simulink subsystem "VehicleBody1DOFLongitudinalSSC"  (R2024a)
settings: Solver=VariableStepAuto  StartTime=0.0  StopTime=10.0  RelTol=1e-3
undefined symbols (not defined in the file): BdyFrm, EnvGrvty, InertFrm, PlntVehCGHgtAxl, PlntVehHtchDst, PlntVehHtchHgtAxl, PlntVehHtchLatDst, PlntWhlLdRadius
libraries: nesl_utility_internal x5, sdl_lib x1
settings Model: ModifiedByFormat=The MathWorks, Inc.  Creator=The MathWorks, Inc.  LastModifiedBy=The MathWorks, Inc.
settings OptimizationCC: ReuseModelBlockBuffer=off
settings DebuggingCC: SubsystemReferenceDiagnosticForUnitTest=warning
settings RTWCC: GPUComputeCapability=3.5

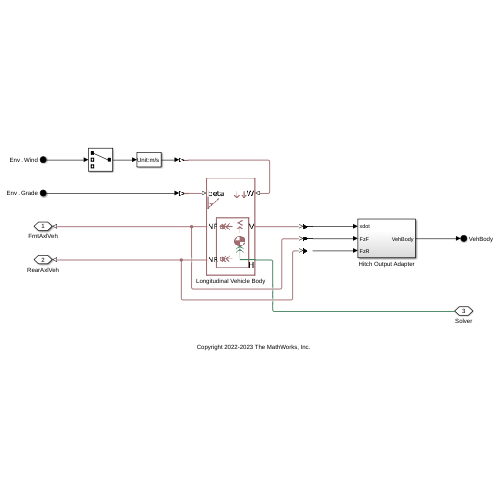
[thumbnail: Simulink's stored preview of the top-level diagram]
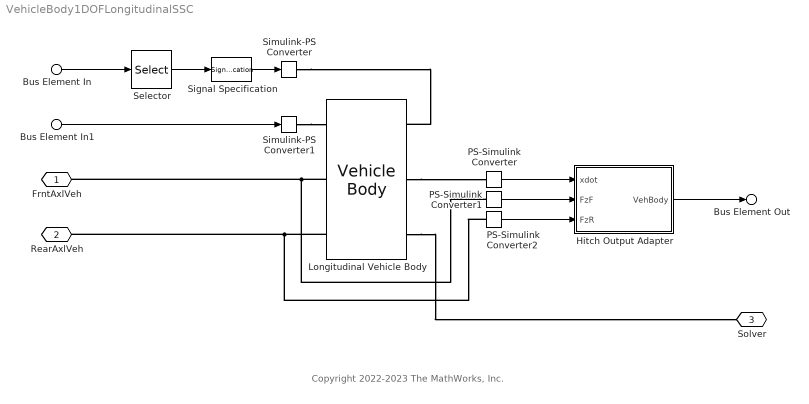
== system VehicleBody1DOFLongitudinalSSC ==
  note: Copyright 2022-2023 The MathWorks, Inc.
  Bus Element In : Inport  PortName=Env  Element=Wind
  Bus Element In1 : Inport  PortName=Env  Element=Grade
  Hitch Output Adapter : Subsystem
  Longitudinal Vehicle Body : sdl_lib/Tires & Vehicles/Vehicle Body  mass=PlntVehMass kg  n_w=PlntVehNumWhlFrntAxl  x_f=PlntVehDstCGFrntAxl m  x_r=PlntVehDstCGRearAxl m  y_c=PlntVehCGHgtAxl+PlntWhlLdRadius m  mass_var=simscape.enum.onoff.off  g=EnvGrvty m/s^2  liftoff_warning=simscape.enum.onoff.off  area=PlntVehAeroFrntArea m^2  Cd=PlntVehAeroDragCff  rho=EnvAirDen kg/m^3  model_pitch=simscape.enum.onoff.off  inertia=PlntVehPitchMomentInertia kg*m^2  suspension_model=sdl.enum.linearTLU.linear  k_f=PlntVeh3DOFFrntSuspStiff N/m  b_f=PlntVeh3DOFFrntSuspDamp N*s/m  k_r=PlntVeh3DOFRearSuspStiff N/m  b_r=PlntVeh3DOFRearSuspDamp N*s/m  k_f_TLU=[-2000, -1000, 0, 1000, 2000] N  x_f_TLU=[-.4, -.2, 0, .2, .4] m  b_f_TLU=[-200, -100, 0, 100, 200] N  v_f_TLU=[-4, -2, 0, 2, 4] m/s  k_r_TLU=[-2000, -1000, 0, 1000, 2000] N  x_r_TLU=[-.4, -.2, 0, .2, .4] m  b_r_TLU=[-200, -100, 0, 100, 200] N  v_r_TLU=[-4, -2, 0, 2, 4] m/s  interp_method=simscape.enum.interpolation.linear  extrap_method=simscape.enum.extrapolation.linear  model_hardstop=simscape.enum.onoff.off  upper_bound_f=.25 m  lower_bound_f=-.25 m  stop_k_f=1e6 N/m  stop_b_f=150 N*s/m  upper_bound_r=.25 m  lower_bound_r=-.25 m  stop_k_r=1e6 N/m  stop_b_r=150 N*s/m  initial_pitch=PlntVehInitPitchAng rad  initial_pitch_rate=PlntVehInitPitchRate rad/s  v_specify=off  v_priority=High  v=0 m/s  v_nominal_specify=off  v_nominal_value=1  v_nominal_unit=m/s
  PS-Simulink Converter : nesl_utility_internal/PS-Simulink Converter  PhysicalDomain=network_engine_domain  SubClassName=ps_output  LeftPortType=input  RightPortType=output  PseudoPeriodic=off  Frequencies=[]  VectorFormat=inherit  Unit=inherit  AffineConversion=off
  PS-Simulink Converter1 : nesl_utility_internal/PS-Simulink Converter  PhysicalDomain=network_engine_domain  SubClassName=ps_output  LeftPortType=input  RightPortType=output  PseudoPeriodic=off  Frequencies=[]  VectorFormat=inherit  Unit=inherit  AffineConversion=off
  PS-Simulink Converter2 : nesl_utility_internal/PS-Simulink Converter  PhysicalDomain=network_engine_domain  SubClassName=ps_output  LeftPortType=input  RightPortType=output  PseudoPeriodic=off  Frequencies=[]  VectorFormat=inherit  Unit=inherit  AffineConversion=off
  Selector : Selector  InputPortWidth=3  IndexOptions=Index vector (dialog)  Indices=[1]  OutputSizes=1
  Signal Specification : SignalSpecification  Unit=m/s
  Simulink-PS Converter : nesl_utility_internal/Simulink-PS Converter  PhysicalDomain=network_engine_domain  SubClassName=ps_input  LeftPortType=input  RightPortType=output  PseudoPeriodic=off  Frequencies=[]  NoiseDistribution=none  NoiseParameters=[]  Unit=m/s  AffineConversion=off  FilteringAndDerivatives=provide  SimscapeFilterOrder=1  InputFilterTimeConstant=0.001  UdotUserProvided=0
  Simulink-PS Converter1 : nesl_utility_internal/Simulink-PS Converter  PhysicalDomain=network_engine_domain  SubClassName=ps_input  LeftPortType=input  RightPortType=output  PseudoPeriodic=off  Frequencies=[]  NoiseDistribution=none  NoiseParameters=[]  Unit=deg  AffineConversion=off  FilteringAndDerivatives=provide  SimscapeFilterOrder=1  InputFilterTimeConstant=0.001  UdotUserProvided=0
  FrntAxlVeh : PMIOPort  Side=Left
  RearAxlVeh : PMIOPort  Port=2  Side=Left
  Solver : PMIOPort  Port=3  Side=Right
  Bus Element Out : Outport  PortName=VehBody
  wires:
  Bus Element In/1 -> Selector/1
  PS-Simulink Converter/1 -> Hitch Output Adapter/1(xdot)
  Selector/1 -> Signal Specification/1
  Bus Element In1/1 -> Simulink-PS Converter1/1
  PS-Simulink Converter2/1 -> Hitch Output Adapter/3(FzR)
  PS-Simulink Converter1/1 -> Hitch Output Adapter/2(FzF)
  Signal Specification/1 -> Simulink-PS Converter/1
  Hitch Output Adapter/1(VehBody) -> Bus Element Out/1
  connections:
  Longitudinal Vehicle Body/RConn2 -- PS-Simulink Converter1/LConn1 -- FrntAxlVeh/RConn1
  Longitudinal Vehicle Body/RConn1 -- PS-Simulink Converter2/LConn1 -- RearAxlVeh/RConn1
  Longitudinal Vehicle Body/LConn2 -- PS-Simulink Converter/LConn1
  Longitudinal Vehicle Body/LConn1 -- Solver/RConn1
  Simulink-PS Converter/RConn1 -- Longitudinal Vehicle Body/LConn3
  Simulink-PS Converter1/RConn1 -- Longitudinal Vehicle Body/RConn3

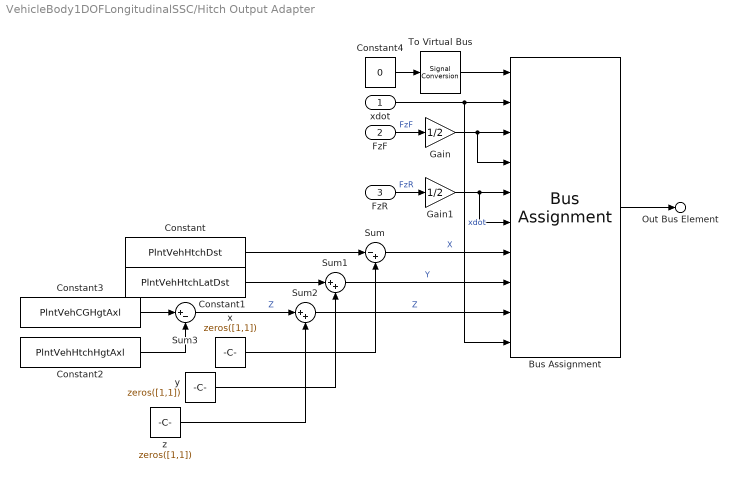
== system VehicleBody1DOFLongitudinalSSC/Hitch Output Adapter ==
  xdot : Inport
  FzF : Inport  Port=2
  FzR : Inport  Port=3
  Bus Assignment : BusAssignment  AssignedSignals=BdyFrm.Cg.Vel.xdot,BdyFrm.Forces.FrntAxl.Lft.Fz,BdyFrm.Forces.FrntAxl.Rght.Fz,BdyFrm.Forces.RearAxl.Lft.Fz,BdyFrm.Forces.RearAxl.Rght.Fz,InertFrm.Hitch.Disp.X,InertFrm.Hitch.Disp.Y,InertFrm.Hitch.Disp.Z,InertFrm.Hitch.Vel.Xdot
  Constant : Constant  Value=PlntVehHtchDst  SampleTime=-1
  Constant1 : Constant  Value=PlntVehHtchLatDst  SampleTime=-1
  Constant2 : Constant  Value=PlntVehHtchHgtAxl  SampleTime=-1
  Constant3 : Constant  Value=PlntVehCGHgtAxl  SampleTime=-1
  Constant4 : Constant  Value=0  OutDataTypeStr=Bus: VehBodyBUS  SampleTime=Inf
  Gain : Gain  Gain=1/2
  Gain1 : Gain  Gain=1/2
  Sum : Sum  Inputs=|-+
  Sum1 : Sum  Inputs=|++
  Sum2 : Sum  Inputs=|++
  Sum3 : Sum  Inputs=|+-
  To Virtual Bus : SignalConversion  ConversionOutput=Virtual bus  OverrideOpt=off
  x : Constant  Value=zeros([1,1])  SampleTime=-1
  y : Constant  Value=zeros([1,1])  SampleTime=-1
  z : Constant  Value=zeros([1,1])  SampleTime=-1
  Out Bus Element : Outport  PortName=VehBody
  wires:
  To Virtual Bus/1 -> Bus Assignment/1
  Bus Assignment/1 -> Out Bus Element/1
  Gain1/1 -> Bus Assignment/5, Bus Assignment/6
  Gain/1 -> Bus Assignment/3, Bus Assignment/4
  FzR/1 -> Gain1/1  "FzR"
  FzF/1 -> Gain/1  "FzF"
  xdot/1 -> Bus Assignment/2, Bus Assignment/10  "xdot"
  Constant4/1 -> To Virtual Bus/1
  z/1 -> Sum2/2
  x/1 -> Sum/2
  y/1 -> Sum1/2
  Constant/1 -> Sum/1
  Sum3/1 -> Sum2/1  "Z"
  Constant3/1 -> Sum3/1
  Sum2/1 -> Bus Assignment/9  "Z"
  Constant2/1 -> Sum3/2
  Sum/1 -> Bus Assignment/7  "X"
  Sum1/1 -> Bus Assignment/8  "Y"
  Constant1/1 -> Sum1/1
